simulink model "jianhua_PMSM_FOC"  (R2025a)
settings: Solver=ode3  StartTime=0.0  StopTime=1  FixedStep=1e-6  RelTol=1e-3
libraries: spsDCVoltageSourceLib x1, spsGroundLib x1, eePmsmFieldOrientedControl x1, spsPermanentMagnetSynchronousMachineLib x1, simulink x1, spsUniversalBridgeLib x1, sps_lib x1
settings Model: Creator=lmh  LastModifiedBy=lmh

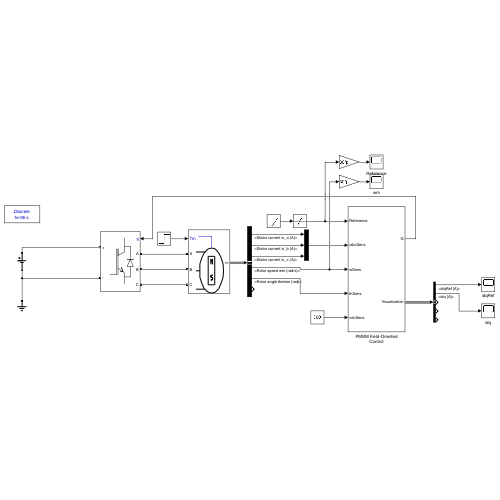
[thumbnail: Simulink's stored preview of the top-level diagram]
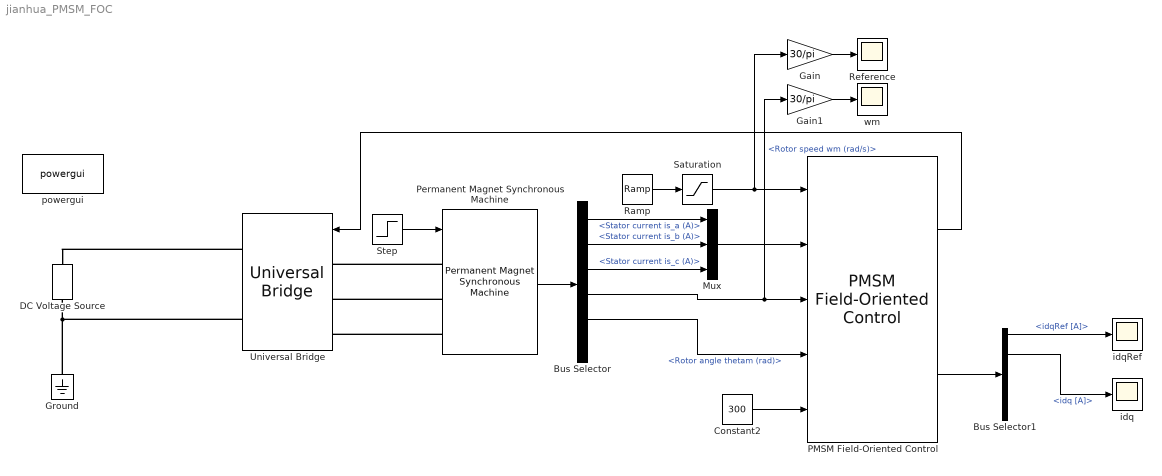
== system jianhua_PMSM_FOC ==
  Bus Selector : BusSelector  OutputSignals=Stator current is_a (A),Stator current is_b (A),Stator current is_c (A),Rotor speed wm (rad/s),Rotor angle thetam (rad),Electromagnetic torque Te (N*m)
  Bus Selector1 : BusSelector  OutputSignals=idqRef [A],idq [A],vdqRef [V],TqRef [N*m],Reference
  Constant2 : Constant  Value=300
  DC Voltage Source : spsDCVoltageSourceLib/DC Voltage Source  Amplitude=300  Measurements=None
  Gain : Gain  Gain=30/pi
  Gain1 : Gain  Gain=30/pi
  Ground : spsGroundLib/Ground  LConnTagsString=a
  Mux : Mux  Inputs=3
  PMSM Field-Oriented Control : eePmsmFieldOrientedControl/PMSM Field-Oriented Control  winding_type=Wye-wound  CtrlMode=Velocity control  Vnom=300  Pmax=1000  Tmax=5  p=4  Vdc_on=50  Ts=1e-6  Tsc=1e-4  CtrlType=PI control  Kp_w=0.05  Ki_w=1  Kv_w=1  Kaw_w=1  RefType=Zero d-axis control  rpmVec=[0, 3000]  TqVec=[-100, 0, 100]  VdcVec=[300, 350]  PWMMode=SVM: space vector modulation  ModFactor=1  idMatrix=zeros(2,3,2)  iqMatrix=zeros(2,3,2)  psim=0.04  Ld=0.00024  Lq=0.00029  Rs=0.01  AxisAlignment=Q-axis  Kp_id=4  Ki_id=30  Kaw_id=1  Kp_iq=4  Ki_iq=30  Kaw_iq=1  AxisPrio=Q-axis  ActZC=off  ActFF=on  ParamTypeFF=Constant parameters  LdFF=8.5e-3  LqFF=8.5e-3  psimFF=0.1194  idVect=[-200, 0, 200]  iqVect=[-200, 0, 200]  LdMatrix=0.0002 * ones(3, 3)  LqMatrix=0.0002 * ones(3, 3)  psimMatrix=0.04 * ones(3, 3)  CPWMMode=SVM: space vector modulation  fsw=10000
      settings: LibrarySourceBlock=|
      | ee_sl_lib/PMSM Control/PMSM Field-Oriented
      | Control
  Permanent Magnet Synchronous Machine : spsPermanentMagnetSynchronousMachineLib/Permanent Magnet Synchronous Machine  NbPhases=3  FluxDistribution=Sinusoidal  RotorType=Round  MechanicalLoad=Torque Tm  PresetModel=No  ShowDetailedParameters=on  MeasurementBus=off  Resistance=0.0485  Inductance=8.5e-3  dqInductances=[8.5e-3,8.5e-3]  La=8.5e-3  MachineConstant=Flux linkage established by magnets (V.s)  Flux=0.1194  VoltageCst=86.6271  TorqueCst=0.7164  Flat=120  Mechanical=[1e-3 1e-4 4 0]  PolePairs=4  InitialConditions=[0,0, 0,0]  InitialConditions5ph=[0 0 0 0 0 0]  RefAngle=90 degrees behind phase A axis (modified Park)  IterativeDiscreteModel=Trapezoidal non iterative  TsBlock=-1  TsPowergui=0
  Ramp : simulink/Sources/Ramp  slope=157.08  start=0.05  InitialOutput=0
  Reference : Scope
      settings: ActiveDisplayYMinimum=-62.500146152187291  ActiveDisplayYMaximum=562.5013153696857
  Saturation : Saturate  UpperLimit=52.36  LowerLimit=0
  Step : Step  Time=0.5  After=0  SampleTime=1e-6
  Universal Bridge : spsUniversalBridgeLib/Universal Bridge  Arms=3  SnubberResistance=1e5  SnubberCapacitance=inf  Device=IGBT / Diodes  Ron=1e-3  Lon=0  ForwardVoltages="[  0  0  ]"  ForwardVoltage=0  GTOparameters=[ 10e-6 , 20e-6 ]  IGBTparameters=[ 1e-6 , 2e-6 ]  Measurements=None  Measurements_2=None  converterType=Rectifier
  idq : Scope
      settings: ActiveDisplayYMinimum=-0.803012654998282  ActiveDisplayYMaximum=1.1347435588564942  DataLoggingVariableName=ScopeData3
  idqRef : Scope
      settings: ActiveDisplayYMinimum=-0.66172323506059949  ActiveDisplayYMaximum=1.1201522577986966  DataLoggingVariableName=ScopeData2
  powergui : sps_lib/powergui  Priority=1  SimulationMode=Discrete  SampleTime=1e-6  frequency=60  Iterations=50  frequencyindice=0  Pbase=100e6  ErrMax=1e-4  UnitsV=kV  UnitsW=MW  buscounter=0  FunctionMessages=off  echomessages=off  EnableUseOfTLC=off  CurrentSourceSwitches=off  DisableSnubberDevices=off  DisableRonSwitches=off  DisableVfSwitches=off  DisplayEquations=off  AutomaticDiscreteSolvers=off  SolverType=Tustin/Backward Euler (TBE)  Interpol=off  ExternalGateDelay=off  methode=off  Ts=100  x0status=blocks  SPID=on  SwTol=0  HookPort=off  NonlinearTolerance=1e-4  nMaxIteration=100  ContinueOnMaxIteration=off  RestoreLinks=warning  ResistiveCurrentMeasurement=off  Frange=[0:2:500]  Ylog=off  Xlog=on  ShowGrid=off  save=off  variable=ZData  structure=0  ZoomFFT=off  StartTime=0.0  cycles=1  DisplayStyle=1  fundamental=60  FreqAxis=off  MaxFrequency=1000  frequencyindicesteady=1  RmsSteady=1  display=off
  wm : Scope
      settings: ActiveDisplayYMinimum=-63.141716946593604  ActiveDisplayYMaximum=568.27545251934248
  wires:
  Ramp/1 -> Saturation/1
  Permanent Magnet Synchronous Machine/1 -> Bus Selector/1
  Bus Selector/1 -> Mux/1  "<Stator current is_a (A)>"
  Bus Selector/2 -> Mux/2  "<Stator current is_b (A)>"
  Bus Selector/3 -> Mux/3  "<Stator current is_c (A)>"
  Mux/1 -> PMSM Field-Oriented Control/2
  Saturation/1 -> Gain/1, PMSM Field-Oriented Control/1
  Bus Selector/4 -> PMSM Field-Oriented Control/3, Gain1/1  "<Rotor speed wm (rad/s)>"
  Bus Selector/5 -> PMSM Field-Oriented Control/4  "<Rotor angle thetam (rad)>"
  Constant2/1 -> PMSM Field-Oriented Control/5
  PMSM Field-Oriented Control/1 -> Universal Bridge/1
  PMSM Field-Oriented Control/2 -> Bus Selector1/1
  Gain/1 -> Reference/1
  Gain1/1 -> wm/1
  Bus Selector1/1 -> idqRef/1  "<idqRef [A]>"
  Bus Selector1/2 -> idq/1  "<idq [A]>"
  Step/1 -> Permanent Magnet Synchronous Machine/1
  connections:
  Universal Bridge/RConn1 -- DC Voltage Source/RConn1
  Universal Bridge/RConn2 -- Ground/LConn1 -- DC Voltage Source/LConn1
  Permanent Magnet Synchronous Machine/LConn2 -- Universal Bridge/LConn2
  Permanent Magnet Synchronous Machine/LConn3 -- Universal Bridge/LConn3
  Permanent Magnet Synchronous Machine/LConn1 -- Universal Bridge/LConn1
